simulink model "plant_block"  (R2019b)
settings: Solver=VariableStepAuto  StartTime=0.0  StopTime=10.0  RelTol=1e-3
libraries: simulink x2
settings Model: Creator=Nilpa  LastModifiedBy=Nilpa

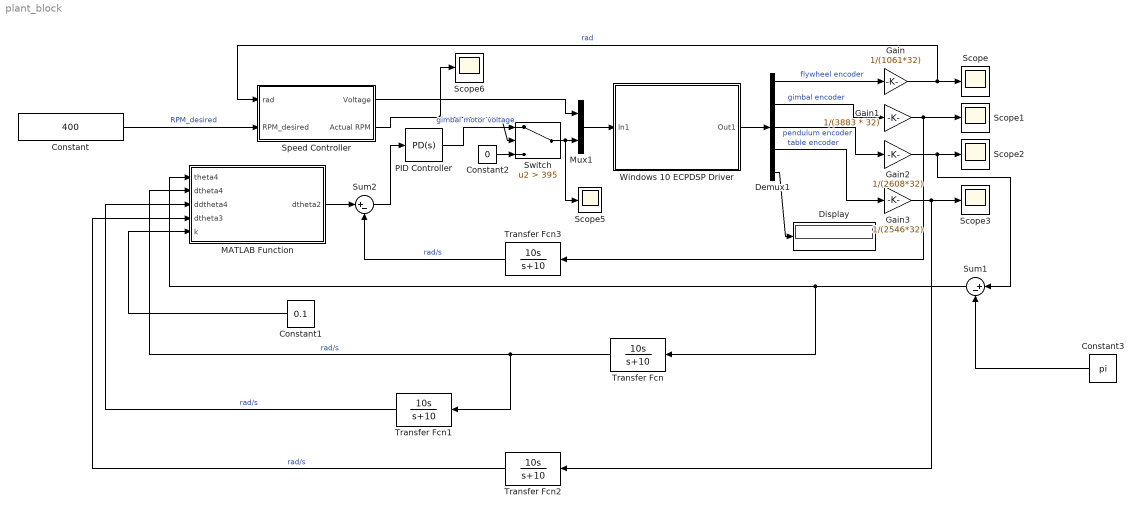
== system plant_block ==
  Constant : Constant  Value=400
  Constant1 : Constant  Value=0.1
  Constant2 : Constant  Value=0
  Constant3 : Constant  Value=pi
  Demux1 : Demux  Outputs=5
  Display : Display
  Gain : Gain  Gain=1/(1061*32)
  Gain1 : Gain  Gain=1/(3883 * 32)
  Gain2 : Gain  Gain=1/(2608*32)
  Gain3 : Gain  Gain=1/(2546*32)
  MATLAB Function : MATLAB Function  TreatAsAtomicUnit=on
  Mux1 : Mux  Inputs=2
  PID Controller : simulink/Continuous/PID Controller  Controller=PD  Form=Parallel  TimeDomain=Continuous-time  SampleTime=-1  IntegratorMethod=Forward Euler  FilterMethod=Forward Euler  ControllerParametersSource=internal  P=1500  I=0  D=38  UseFilter=on  N=100  TunerSelectOption=Transfer Function Based (PID Tuner App)  InitialConditionSource=internal  InitialConditionForIntegrator=0  InitialConditionForFilter=0  DifferentiatorICPrevScaledInput=0  ExternalReset=none  TrackingMode=off  Kt=1  LimitOutput=off  UpperSaturationLimit=inf  LowerSaturationLimit=-inf  LinearizeAsGain=on  AntiWindupMode=none  Kb=1  POutMin=[]  POutMax=[]  IOutMin=[]  IOutMax=[]  DOutMin=[]  DOutMax=[]  NOutMin=[]  NOutMax=[]  SumOutMin=[]  SumOutMax=[]  SaturationOutMin=[]  SaturationOutMax=[]  PParamMin=[]  PParamMax=[]  IParamMin=[]  IParamMax=[]  DParamMin=[]  DParamMax=[]  NParamMin=[]  NParamMax=[]  KbParamMin=[]  KbParamMax=[]  KtParamMin=[]  KtParamMax=[]  KbOutMin=[]  KbOutMax=[]  KtOutMin=[]  KtOutMax=[]  IntegratorOutMin=[]  IntegratorOutMax=[]  FilterOutMin=[]  FilterOutMax=[]  SumI1OutMin=[]  SumI1OutMax=[]  SumI2OutMin=[]  SumI2OutMax=[]  SumI3OutMin=[]  SumI3OutMax=[]  SumI4OutMin=[]  SumI4OutMax=[]  SumDOutMin=[]  SumDOutMax=[]  DifferentiatorOutMin=[]  DifferentiatorOutMax=[]  FilterDiffOutCoefMin=[]  FilterDiffOutCoefMax=[]  ReciprocalOutMin=[]  ReciprocalOutMax=[]  SumDenOutMin=[]  SumDenOutMax=[]  SumNumOutMin=[]  SumNumOutMax=[]  DivideOutMin=[]  DivideOutMax=[]  IntegratorContinuousStateAttributes=''  IntegratorStateMustResolveToSignalObject=off  IntegratorRTWStateStorageClass=Auto  FilterContinuousStateAttributes=''  FilterStateMustResolveToSignalObject=off  FilterRTWStateStorageClass=Auto  ParallelPVariant=InternalParameters  IdealPVariant=Disabled  IVariant=Disabled  DVariant=InternalParameters  IntegratorVariant=Disabled  SatVariant=Disabled  AWVariant=Disabled  PCopyVariant=Disabled  TRVariant=Disabled  FdbkBlocksVariant=Forward  IdealPFdbkVariant=Disabled  SatFdbkVariant=Disabled  DerivativeFilterVariant=ContFilter  NVariant=InternalParameters  NCopyVariant=Disabled  FilterICVariant=InternalICsFilter  IntegratorICVariant=Disabled  ExternalResetVariant=Disabled  TRSumVariant=Passthrough  SumFdbkVariant=Disabled  SumVariant=Sum_PD
  Scope{,1..3,5..6} (6 alike) : Scope
  "Speed Controller " : Subsystem
  Sum1 : Sum  Inputs=|+-
  Sum2 : Sum  Inputs=|+-
  Switch : Switch  Criteria=u2 > Threshold  Threshold=395
  Transfer Fcn{,1..3} (4 alike) : TransferFcn  Numerator=[10 0 ]  Denominator=[1 10]
  Windows 10 ECPDSP Driver : Subsystem  mask{BaseAddr='0x3F00', STime=0.008, TimeOutPer=500, HWAccess=on}
      mask prompts: BaseAddr "Base I/O Address"; STime "Sample Time (Sec)"; TimeOutPer "Timeout Period (500 ~ 2000)"; HWAccess "Hardware Access"
      mask Display: color('black');disp('ECPDSP Driver\n upto\n 4 Encs(ADC Channels)\n and 2 Dacs')
  wires:
  Demux1/2 -> Gain1/1  "gimbal encoder"
  Gain2/1 -> Scope2/1, Sum1/1
  Constant2/1 -> Switch/3
  Sum1/1 -> MATLAB Function/1(theta4), Transfer Fcn/1
  Gain/1 -> "Speed Controller "/1(rad), Scope/1  "rad"
  Demux1/4 -> Gain3/1  "table encoder"
  Switch/1 -> Scope5/1, Mux1/2
  Constant/1 -> "Speed Controller "/2(RPM_desired)  "RPM_desired"
  Constant3/1 -> Sum1/2
  Transfer Fcn/1 -> Transfer Fcn1/1, MATLAB Function/2(dtheta4)  "rad/s"
  Gain1/1 -> Transfer Fcn3/1, Scope1/1
  Demux1/5 -> Display/1
  Constant1/1 -> MATLAB Function/5(k)
  "Speed Controller "/2("Actual RPM ") -> Scope6/1, Switch/2
  PID Controller/1 -> Switch/1  "gimbal motor voltage"
  Demux1/3 -> Gain2/1  "pendulum encoder"
  Demux1/1 -> Gain/1  "flywheel encoder"
  "Speed Controller "/1(Voltage) -> Mux1/1
  Gain3/1 -> Transfer Fcn2/1, Scope3/1
  Windows 10 ECPDSP Driver/1(Out1) -> Demux1/1
  Mux1/1 -> Windows 10 ECPDSP Driver/1(In1)
  Transfer Fcn1/1 -> MATLAB Function/3(ddtheta4)  "rad/s"
  Transfer Fcn2/1 -> MATLAB Function/4(dtheta3)  "rad/s"
  MATLAB Function/1(dtheta2) -> Sum2/1
  Sum2/1 -> PID Controller/1
  Transfer Fcn3/1 -> Sum2/2  "rad/s"

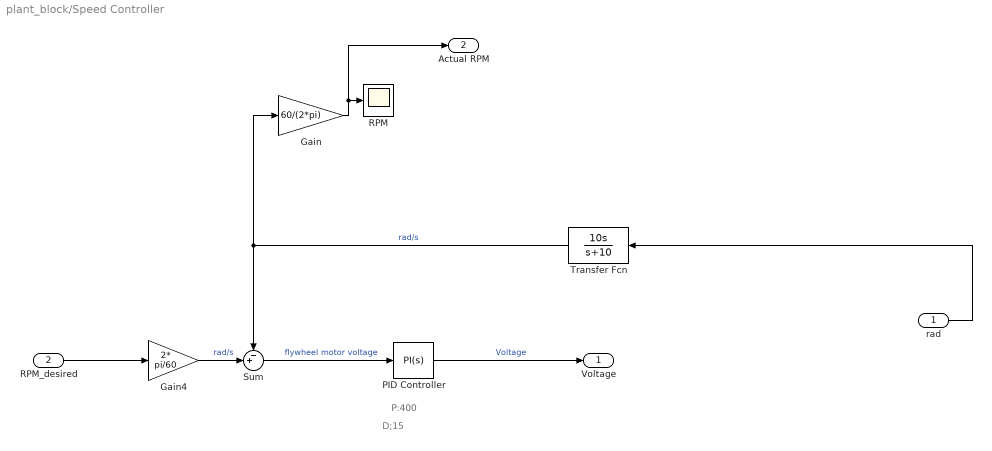
== system plant_block/Speed Controller  ==
  note: D;15
  note: P:400
  rad : Inport
  RPM_desired : Inport  Port=2
  Gain : Gain  Gain=60/(2*pi)
  Gain4 : Gain  Gain=2* pi/60
  PID Controller : simulink/Continuous/PID Controller  Controller=PI  Form=Parallel  TimeDomain=Continuous-time  SampleTime=-1  IntegratorMethod=Forward Euler  FilterMethod=Forward Euler  ControllerParametersSource=internal  P=400  I=15  D=0  UseFilter=on  N=100  TunerSelectOption=Transfer Function Based (PID Tuner App)  InitialConditionSource=internal  InitialConditionForIntegrator=0  InitialConditionForFilter=0  DifferentiatorICPrevScaledInput=0  ExternalReset=none  TrackingMode=off  Kt=1  LimitOutput=off  UpperSaturationLimit=inf  LowerSaturationLimit=-inf  LinearizeAsGain=on  AntiWindupMode=none  Kb=1  POutMin=[]  POutMax=[]  IOutMin=[]  IOutMax=[]  DOutMin=[]  DOutMax=[]  NOutMin=[]  NOutMax=[]  SumOutMin=[]  SumOutMax=[]  SaturationOutMin=[]  SaturationOutMax=[]  PParamMin=[]  PParamMax=[]  IParamMin=[]  IParamMax=[]  DParamMin=[]  DParamMax=[]  NParamMin=[]  NParamMax=[]  KbParamMin=[]  KbParamMax=[]  KtParamMin=[]  KtParamMax=[]  KbOutMin=[]  KbOutMax=[]  KtOutMin=[]  KtOutMax=[]  IntegratorOutMin=[]  IntegratorOutMax=[]  FilterOutMin=[]  FilterOutMax=[]  SumI1OutMin=[]  SumI1OutMax=[]  SumI2OutMin=[]  SumI2OutMax=[]  SumI3OutMin=[]  SumI3OutMax=[]  SumI4OutMin=[]  SumI4OutMax=[]  SumDOutMin=[]  SumDOutMax=[]  DifferentiatorOutMin=[]  DifferentiatorOutMax=[]  FilterDiffOutCoefMin=[]  FilterDiffOutCoefMax=[]  ReciprocalOutMin=[]  ReciprocalOutMax=[]  SumDenOutMin=[]  SumDenOutMax=[]  SumNumOutMin=[]  SumNumOutMax=[]  DivideOutMin=[]  DivideOutMax=[]  IntegratorContinuousStateAttributes=''  IntegratorStateMustResolveToSignalObject=off  IntegratorRTWStateStorageClass=Auto  FilterContinuousStateAttributes=''  FilterStateMustResolveToSignalObject=off  FilterRTWStateStorageClass=Auto  ParallelPVariant=InternalParameters  IdealPVariant=Disabled  IVariant=InternalParameters  DVariant=Disabled  IntegratorVariant=Continuous  SatVariant=Disabled  AWVariant=Passthrough  PCopyVariant=Disabled  TRVariant=Disabled  FdbkBlocksVariant=Forward  IdealPFdbkVariant=Disabled  SatFdbkVariant=Disabled  DerivativeFilterVariant=Disabled  NVariant=Disabled  NCopyVariant=Disabled_SignalSpec  FilterICVariant=Disabled  IntegratorICVariant=InternalICs  ExternalResetVariant=Disabled  TRSumVariant=Passthrough  SumFdbkVariant=Disabled  SumVariant=Sum_PI
  RPM : Scope
  Sum : Sum  Inputs=-+|
  Transfer Fcn : TransferFcn  Numerator=[10 0 ]  Denominator=[1 10]
  Voltage : Outport
  "Actual RPM " : Outport  Port=2
  wires:
  Gain4/1 -> Sum/2  "rad/s"
  Transfer Fcn/1 -> Gain/1, Sum/1  "rad/s"
  Sum/1 -> PID Controller/1  "flywheel motor voltage"
  PID Controller/1 -> Voltage/1  "Voltage"
  RPM_desired/1 -> Gain4/1
  rad/1 -> Transfer Fcn/1
  Gain/1 -> "Actual RPM "/1, RPM/1

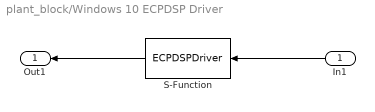
== system plant_block/Windows 10 ECPDSP Driver ==
  In1 : Inport
  S-Function : S-Function  FunctionName=ECPDSPDriver  Parameters=BaseAddr,STime,TimeOutPer,HWAccess  SFunctionDeploymentMode=off  EnableBusSupport=off
  Out1 : Outport
  wires:
  In1/1 -> S-Function/1
  S-Function/1 -> Out1/1

== matlab function plant_block/MATLAB Function ==
  data: theta4 input; dtheta2 output; dtheta4 input; ddtheta4 input; dtheta3 input; k input
function dtheta2 = fcn(theta4, dtheta4, ddtheta4, dtheta3, k)
m = 0.1580;
lcg = 0.2698;
rh = 0.37;
J1 = 0.1314;
Jz_bar = 0.0131;
g = 9.81;
c = 0.2;
Eo = 0;
Id = 0.0148;
dtheta1 = 400 * (2*pi/60);

E = 0.5*m*lcg^2*dtheta4^2 + m*g*lcg*(cos(theta4) - 1);

% might need to negate k...simulation says so...???
ddtheta3 = -k*(E - Eo)*dtheta4*cos(theta4);

dtheta2 = (rh/(Id*dtheta1))*...
    ((J1+m*rh^2)*ddtheta3 + m*lcg*rh*cos(theta4)*ddtheta4 - ...
    m*lcg*rh*sin(theta4)*dtheta4^2 + c*dtheta3);
end
